simulink model "open_loop_SHITY"  (R2019a)
settings: Solver=FixedStepAuto  StartTime=0.0  StopTime=10.0  FixedStep=1/100  RelTol=1e-3  AbsTol=1e-3
model workspace: external: MATLAB File params.m (data not in the file)
values from neighbouring files (symbols this model uses):
  b = 2.75e-11    [help_linearize.m]
  k = 1e-9    (= 1e-09)    [help_linearize.m]
undefined symbols (not defined in the file or in its folder): g, m
libraries: nesl_utility x9
settings Model: Creator=Jocke  LastModifiedBy=Stefan
settings SolverCC: AutoScaleAbsTol=off
settings DataIOCC: SaveState=on  ReturnWorkspaceOutputs=off
settings DebuggingCC: ArithmeticOperatorsInVariantConditions=warning
settings SFSimCC: SimUseLocalCustomCode=off
settings RTWCC: RTWUseLocalCustomCode=off
settings CodeAppCC: StateflowObjectComments=on
settings SimscapeCC: SimscapeNormalizeSystem=off  SimscapeLogType=all  SimscapeLogDataHistory=10000

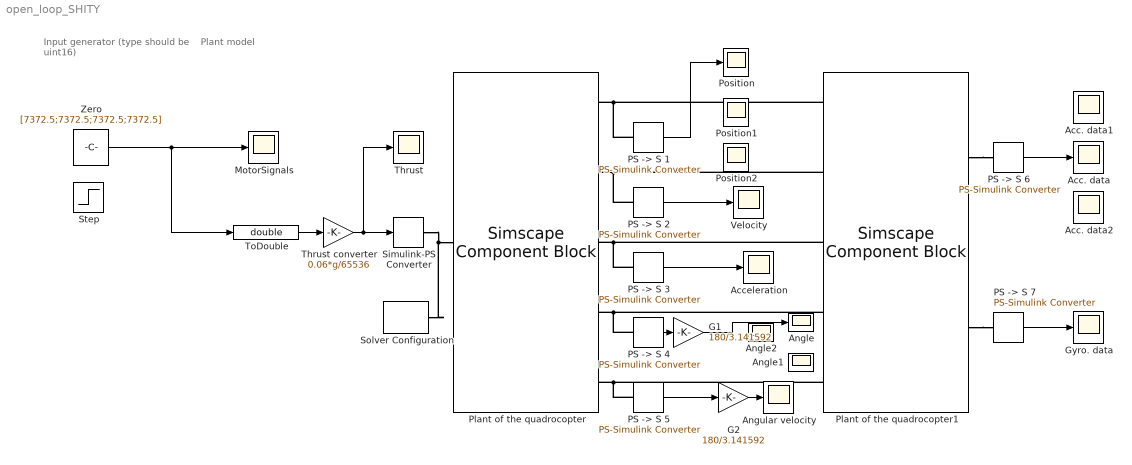
== system open_loop_SHITY ==
  note: Input generator
      | (type should be uint16)
  note: Plant model
  Acc. data : Scope
  Acc. data1 : Scope
  Acc. data2 : Scope
  Acceleration : Scope
  Angle : Scope
  Angle1 : Scope
  Angle2 : Scope
  Angular velocity : Scope
  G1 : Gain  Gain=180/3.141592
  G2 : Gain  Gain=180/3.141592
  Gyro. data : Scope
  MotorSignals : Scope
  PS -> S {1..7} (7 alike) : nesl_utility/PS-Simulink Converter  PhysicalDomain=network_engine_domain  SubClassName=ps_output  LeftPortType=input  RightPortType=output  PseudoPeriodic=off  Frequencies=[]  Unit=1  AffineConversion=off
  Plant of the quadrocopter : SimscapeComponentBlock  SourceFile=plant  ComponentPath=plant  ComponentVariants=plant  ComponentVariantNames=plant  ClassName=plant  SchemaVersion=1  m=m kg  g=g m/s^2  d=d m  k=k  b=b  unit=1 m
      settings: CopyFcn=simscape.engine.sli.internal.componentblockcallback(gcbh,'COPY')  PreCopyFcn=simscape.engine.sli.internal.componentblockcallback(gcbh,'PRECOPY')  PreDeleteFcn=simscape.engine.sli.internal.componentblockcallback(gcbh,'PREDELETE')
      mask Type: Plant of quadrocopter
  Plant of the quadrocopter1 : SimscapeComponentBlock  SourceFile=sensors  ComponentPath=sensors  ComponentVariants=sensors  ComponentVariantNames=sensors  ClassName=sensors  SchemaVersion=1  m=m kg  g=g m/s^2  d=d m  k=k  b=b
      settings: CopyFcn=simscape.engine.sli.internal.componentblockcallback(gcbh,'COPY')  PreCopyFcn=simscape.engine.sli.internal.componentblockcallback(gcbh,'PRECOPY')  PreDeleteFcn=simscape.engine.sli.internal.componentblockcallback(gcbh,'PREDELETE')
      mask Type: Plant of quadrocopter
  Position : Scope
  Position1 : Scope
  Position2 : Scope
  Simulink-PS Converter : nesl_utility/Simulink-PS Converter  PhysicalDomain=network_engine_domain  SubClassName=ps_input  LeftPortType=input  RightPortType=output  PseudoPeriodic=off  Frequencies=[]  NoiseDistribution=none  NoiseParameters=[]  Unit=1  AffineConversion=off  FilteringAndDerivatives=zero  SimscapeFilterOrder=1  InputFilterTimeConstant=0.001  UdotUserProvided=1
  Solver Configuration : nesl_utility/Solver Configuration  PhysicalDomain=network_engine_domain  SubClassName=solver  LeftPortType=input  RightPortType=generic  Tones=[]  Harmonics=[]  SimulateNoise=off  Profile=off  UseLocalSampling=off  EnableSwitchedLinearOptims=on  FrequencyDomain=off  UseCCode=off  RelTol=0.001  AbsTol=1e-06  MinStep=1e-09  ToWorkspace=off  RevertToSquareIcSolve=off  NumHomotopyIterations=100  PhasorMode=off  PhasorModeNumHarmonics=1  DoDC=on  ResidualTolerance=1e-09  UseLocalSolver=off  LocalSolverChoice=NE_BACKWARD_EULER_ADVANCER  LocalSolverSampleTime=0.001  DoFixedCost=off  MaxNonlinIter=3  MaxModeIter=2  LinearAlgebra=Sparse  EquationFormulation=NE_TIME_EF  DelaysMemoryBudget=1024  AutomaticFiltering=on  FilteringTimeConstant=0.001  PartitionStorageMethod=AS_NEEDED  PartitionMemoryBudget=1024  PartitionMethod=FAST
  Step : Step  Time=[4; 0; 6; 0]  Before=[0; 0; 0; 0]  After=[1000; 0; 2000; 0]  SampleTime=0
  Thrust : Scope
  Thrust converter : Gain  Gain=0.06*g/65536
  ToDouble : DataTypeConversion  OutDataTypeStr=double  RndMeth=Round  SaturateOnIntegerOverflow=on
  Velocity : Scope
  Zero : Constant  Value=[7372.5;7372.5;7372.5;7372.5]  VectorParams1D=off  OutDataTypeStr=uint16
  wires:
  "PS -> S 7"/1 -> Gyro. data/1
  G2/1 -> Angular velocity/1
  ToDouble/1 -> Thrust converter/1
  Thrust converter/1 -> Thrust/1, Simulink-PS Converter/1
  "PS -> S 5"/1 -> G2/1
  "PS -> S 4"/1 -> G1/1
  "PS -> S 3"/1 -> Acceleration/1
  "PS -> S 2"/1 -> Velocity/1
  "PS -> S 1"/1 -> Position/1
  G1/1 -> Angle/1
  Zero/1 -> ToDouble/1, MotorSignals/1
  "PS -> S 6"/1 -> Acc. data/1
  connections:
  Plant of the quadrocopter/LConn1 -- Simulink-PS Converter/RConn1 -- Solver Configuration/RConn1
  Plant of the quadrocopter/RConn1 -- Plant of the quadrocopter1/LConn1 -- "PS -> S 1"/LConn1
  Plant of the quadrocopter/RConn2 -- Plant of the quadrocopter1/LConn2 -- "PS -> S 2"/LConn1
  Plant of the quadrocopter/RConn3 -- Plant of the quadrocopter1/LConn3 -- "PS -> S 3"/LConn1
  Plant of the quadrocopter/RConn4 -- Plant of the quadrocopter1/LConn4 -- "PS -> S 4"/LConn1
  Plant of the quadrocopter/RConn5 -- Plant of the quadrocopter1/LConn5 -- "PS -> S 5"/LConn1
  Plant of the quadrocopter1/RConn1 -- "PS -> S 6"/LConn1
  Plant of the quadrocopter1/RConn2 -- "PS -> S 7"/LConn1
